simulink model "ALL_JP360_DBW_V6_5_1103"  (R2022a)
settings: Solver=FixedStepAuto  StartTime=0.0  StopTime=inf  FixedStep=0.01  RelTol=1e-3  EnableMultiTasking=on
model workspace (MAT data in the model file):
  g = 9.8
undefined symbols (not defined in the file or in its folder): canChannel, delta_v_p, IPM_Line_C0, IPM_Line_C1, IPM_Line_C2, IPM_Line_C3, M, M_p, MRR_ObjDistX, MRR_ObjDistY, MRR_ObjFusionCamID, MRR_ObjFusionSig, MRR_ObjID, MRR_ObjRelVelX, MRR_ObjRelVelY, MRR_ObjType, MRR_ObjUpdFlg, none, obj_vaild, untracktime, V, videoinput
libraries: canfdmsglib x230, canfdlib x76, slpidlib x24, simulink x18, dspstat3 x14, ctrlSharedLib x1, simulink_extras x1, imaqlib x1, realtime_pacer_lib x1, dspvision x1, visionsinks x1
(part 42 of 55)

== system ALL_JP360_DBW_V6_5_1103/MsgFromCAN/VR_ADCU_MsgFromCAN/VR_ADCU_IPM_Line_01_0x640 ==
  VR_ADCU_IPM_Line_01_0x640FromInData : Inport  OutDataTypeStr=Bus:CAN_FD_MESSAGE_BUS
  Bus Creator : BusCreator  Inputs=12  OutDataTypeStr=Bus:VR_ADCU_IPM_Line_01_0x640  NonVirtualBus=on
  CAN FD Unpack : canfdmsglib/CAN FD Unpack  CANdbFile=HiFire_T360_P789_1R1V_Pri_Matrix_CAN_V2.3_20220810.dbc  MsgList=(none)  MsgName=IPM_Line_01_0x640  ProtocolMode=CAN FD  MsgIDType=Standard (11-bit identifier)  MsgIdentifier=1600  MsgLength=20  SignalInfo={'IPM_Line01_BlockCounter','90','11','BE','unsigned','Standard','0','1','0','0','2047';'IPM_Line01_C0','115','13','BE','unsigned','Standard','0','0.0039062','-16','-16','15.9961';'IPM_Line01_C1','61','13','BE','unsigned','Standard','0','0.00048828','-1.6','-1.6','1.6002';'IPM_Line01_C2','65','12','BE','unsigned','Standard','0','1.5259e-05','-0.031243','-0.031243','0.031206';'IPM_Line01_C3','85','12','BE','unsigned','Standard','0','3.8147e-06','-0.0078125','-0.0078125','0.0078087';'IPM_Line01_Checksum','152','16','BE','unsigned','Standard','0','1','0','0','65535';'IPM_Line01_ColorClass','12','3','BE','unsigned','Standard','0','1','0','0','7';'IPM_Line01_Existence_Probability','96','8','BE','unsigned','Standard','0','0.01','0','0','1';'IPM_Line01_MsgCounter','136','4','BE','unsigned','Standard','0','1','0','0','15';'IPM_Line01_Type','15','5','BE','unsigned','Standard','0','1','0','0','31';'IPM_Line01_ViewRangeEnd','37','10','BE','unsigned','Standard','0','0.25','0','0','255.75';'IPM_Line01_ViewRangeStart','31','13','BE','unsigned','Standard','0','0.025','0','0','204.775'}  IDPort=off  TimestampPort=off  ErrorPort=off  RemotePort=off  LengthPort=off  StatusPort=off  BRSPort=off  ESIPort=off  DLCPort=off  ApplyMinMax=off
      settings: SourceProductBaseCode=ME,XP,VN  DataFormat=CANdb specified signals
  Data Type Conversion1 : DataTypeConversion  OutDataTypeStr=int16  SaturateOnIntegerOverflow=off  RndMeth=Floor
  Data Type Conversion10 : DataTypeConversion  OutDataTypeStr=int8  SaturateOnIntegerOverflow=off  RndMeth=Floor
  Data Type Conversion{2..5,8,11..12} (7 alike) : DataTypeConversion  OutDataTypeStr=single  SaturateOnIntegerOverflow=off  RndMeth=Floor
  Data Type Conversion6 : DataTypeConversion  OutDataTypeStr=uint16  SaturateOnIntegerOverflow=off  RndMeth=Floor
  Data Type Conversion7 : DataTypeConversion  OutDataTypeStr=int8  SaturateOnIntegerOverflow=off  RndMeth=Floor
  Data Type Conversion9 : DataTypeConversion  OutDataTypeStr=int8  SaturateOnIntegerOverflow=off  RndMeth=Floor
  VR_ADCU_IPM_Line_01_0x640FromOutData : Outport  OutDataTypeStr=Bus:VR_ADCU_IPM_Line_01_0x640
  wires:
  CAN FD Unpack/1 -> Data Type Conversion1/1
  CAN FD Unpack/2 -> Data Type Conversion2/1
  CAN FD Unpack/3 -> Data Type Conversion3/1
  CAN FD Unpack/4 -> Data Type Conversion4/1
  CAN FD Unpack/5 -> Data Type Conversion5/1
  CAN FD Unpack/6 -> Data Type Conversion6/1
  CAN FD Unpack/7 -> Data Type Conversion7/1
  CAN FD Unpack/8 -> Data Type Conversion8/1
  CAN FD Unpack/9 -> Data Type Conversion9/1
  CAN FD Unpack/10 -> Data Type Conversion10/1
  CAN FD Unpack/11 -> Data Type Conversion11/1
  CAN FD Unpack/12 -> Data Type Conversion12/1
  Data Type Conversion1/1 -> Bus Creator/1  "IPM_Line01_BlockCounter"
  Data Type Conversion2/1 -> Bus Creator/2  "IPM_Line01_C0"
  Data Type Conversion3/1 -> Bus Creator/3  "IPM_Line01_C1"
  Data Type Conversion4/1 -> Bus Creator/4  "IPM_Line01_C2"
  Data Type Conversion5/1 -> Bus Creator/5  "IPM_Line01_C3"
  Data Type Conversion6/1 -> Bus Creator/6  "IPM_Line01_Checksum"
  Data Type Conversion7/1 -> Bus Creator/7  "IPM_Line01_ColorClass"
  Data Type Conversion8/1 -> Bus Creator/8  "IPM_Line01_Existence_Probability"
  Data Type Conversion9/1 -> Bus Creator/9  "IPM_Line01_MsgCounter"
  Data Type Conversion10/1 -> Bus Creator/10  "IPM_Line01_Type"
  Data Type Conversion11/1 -> Bus Creator/11  "IPM_Line01_ViewRangeEnd"
  Data Type Conversion12/1 -> Bus Creator/12  "IPM_Line01_ViewRangeStart"
  Bus Creator/1 -> VR_ADCU_IPM_Line_01_0x640FromOutData/1  "VR_ADCU_IPM_Line_01_0x640FromOutData"
  VR_ADCU_IPM_Line_01_0x640FromInData/1 -> CAN FD Unpack/1  "VR_ADCU_IPM_Line_01_0x640FromInData"

== system ALL_JP360_DBW_V6_5_1103/MsgFromCAN/VR_ADCU_MsgFromCAN/VR_ADCU_IPM_Line_02_0x641 ==
  VR_ADCU_IPM_Line_02_0x641FromInData : Inport  OutDataTypeStr=Bus:CAN_FD_MESSAGE_BUS
  Bus Creator : BusCreator  Inputs=12  OutDataTypeStr=Bus:VR_ADCU_IPM_Line_02_0x641  NonVirtualBus=on
  CAN FD Unpack : canfdmsglib/CAN FD Unpack  CANdbFile=HiFire_T360_P789_1R1V_Pri_Matrix_CAN_V2.3_20220810.dbc  MsgList=(none)  MsgName=IPM_Line_02_0x641  ProtocolMode=CAN FD  MsgIDType=Standard (11-bit identifier)  MsgIdentifier=1601  MsgLength=20  SignalInfo={'IPM_Line02_BlockCounter','90','11','BE','unsigned','Standard','0','1','0','0','2047';'IPM_Line02_C0','115','13','BE','unsigned','Standard','0','0.0039062','-16','-16','15.9961';'IPM_Line02_C1','61','13','BE','unsigned','Standard','0','0.00048828','-1.6','-1.6','1.6002';'IPM_Line02_C2','65','12','BE','unsigned','Standard','0','1.5259e-05','-0.031243','-0.031243','0.031206';'IPM_Line02_C3','85','12','BE','unsigned','Standard','0','3.8147e-06','-0.0078125','-0.0078125','0.0078087';'IPM_Line02_Checksum','152','16','BE','unsigned','Standard','0','1','0','0','65535';'IPM_Line02_ColorClass','12','3','BE','unsigned','Standard','0','1','0','0','7';'IPM_Line02_Existence_Probability','96','8','BE','unsigned','Standard','0','0.01','0','0','1';'IPM_Line02_MsgCounter','136','4','BE','unsigned','Standard','0','1','0','0','15';'IPM_Line02_Type','15','5','BE','unsigned','Standard','0','1','0','0','31';'IPM_Line02_ViewRangeEnd','37','10','BE','unsigned','Standard','0','0.25','0','0','255.75';'IPM_Line02_ViewRangeStart','31','13','BE','unsigned','Standard','0','0.025','0','0','204.775'}  IDPort=off  TimestampPort=off  ErrorPort=off  RemotePort=off  LengthPort=off  StatusPort=off  BRSPort=off  ESIPort=off  DLCPort=off  ApplyMinMax=off
      settings: SourceProductBaseCode=ME,XP,VN  DataFormat=CANdb specified signals
  Data Type Conversion1 : DataTypeConversion  OutDataTypeStr=int16  SaturateOnIntegerOverflow=off  RndMeth=Floor
  Data Type Conversion10 : DataTypeConversion  OutDataTypeStr=int8  SaturateOnIntegerOverflow=off  RndMeth=Floor
  Data Type Conversion{2..5,8,11..12} (7 alike) : DataTypeConversion  OutDataTypeStr=single  SaturateOnIntegerOverflow=off  RndMeth=Floor
  Data Type Conversion6 : DataTypeConversion  OutDataTypeStr=uint16  SaturateOnIntegerOverflow=off  RndMeth=Floor
  Data Type Conversion7 : DataTypeConversion  OutDataTypeStr=int8  SaturateOnIntegerOverflow=off  RndMeth=Floor
  Data Type Conversion9 : DataTypeConversion  OutDataTypeStr=int8  SaturateOnIntegerOverflow=off  RndMeth=Floor
  VR_ADCU_IPM_Line_02_0x641FromOutData : Outport  OutDataTypeStr=Bus:VR_ADCU_IPM_Line_02_0x641
  wires:
  CAN FD Unpack/1 -> Data Type Conversion1/1
  CAN FD Unpack/2 -> Data Type Conversion2/1
  CAN FD Unpack/3 -> Data Type Conversion3/1
  CAN FD Unpack/4 -> Data Type Conversion4/1
  CAN FD Unpack/5 -> Data Type Conversion5/1
  CAN FD Unpack/6 -> Data Type Conversion6/1
  CAN FD Unpack/7 -> Data Type Conversion7/1
  CAN FD Unpack/8 -> Data Type Conversion8/1
  CAN FD Unpack/9 -> Data Type Conversion9/1
  CAN FD Unpack/10 -> Data Type Conversion10/1
  CAN FD Unpack/11 -> Data Type Conversion11/1
  CAN FD Unpack/12 -> Data Type Conversion12/1
  Data Type Conversion1/1 -> Bus Creator/1  "IPM_Line02_BlockCounter"
  Data Type Conversion2/1 -> Bus Creator/2  "IPM_Line02_C0"
  Data Type Conversion3/1 -> Bus Creator/3  "IPM_Line02_C1"
  Data Type Conversion4/1 -> Bus Creator/4  "IPM_Line02_C2"
  Data Type Conversion5/1 -> Bus Creator/5  "IPM_Line02_C3"
  Data Type Conversion6/1 -> Bus Creator/6  "IPM_Line02_Checksum"
  Data Type Conversion7/1 -> Bus Creator/7  "IPM_Line02_ColorClass"
  Data Type Conversion8/1 -> Bus Creator/8  "IPM_Line02_Existence_Probability"
  Data Type Conversion9/1 -> Bus Creator/9  "IPM_Line02_MsgCounter"
  Data Type Conversion10/1 -> Bus Creator/10  "IPM_Line02_Type"
  Data Type Conversion11/1 -> Bus Creator/11  "IPM_Line02_ViewRangeEnd"
  Data Type Conversion12/1 -> Bus Creator/12  "IPM_Line02_ViewRangeStart"
  Bus Creator/1 -> VR_ADCU_IPM_Line_02_0x641FromOutData/1  "VR_ADCU_IPM_Line_02_0x641FromOutData"
  VR_ADCU_IPM_Line_02_0x641FromInData/1 -> CAN FD Unpack/1  "VR_ADCU_IPM_Line_02_0x641FromInData"

== system ALL_JP360_DBW_V6_5_1103/MsgFromCAN/VR_ADCU_MsgFromCAN/VR_ADCU_IPM_Line_03_0x642 ==
  VR_ADCU_IPM_Line_03_0x642FromInData : Inport  OutDataTypeStr=Bus:CAN_FD_MESSAGE_BUS
  Bus Creator : BusCreator  Inputs=12  OutDataTypeStr=Bus:VR_ADCU_IPM_Line_03_0x642  NonVirtualBus=on
  CAN FD Unpack : canfdmsglib/CAN FD Unpack  CANdbFile=HiFire_T360_P789_1R1V_Pri_Matrix_CAN_V2.3_20220810.dbc  MsgList=(none)  MsgName=IPM_Line_03_0x642  ProtocolMode=CAN FD  MsgIDType=Standard (11-bit identifier)  MsgIdentifier=1602  MsgLength=20  SignalInfo={'IPM_Line03_BlockCounter','90','11','BE','unsigned','Standard','0','1','0','0','2047';'IPM_Line03_C0','115','13','BE','unsigned','Standard','0','0.0039062','-16','-16','15.9961';'IPM_Line03_C1','61','13','BE','unsigned','Standard','0','0.00048828','-1.6','-1.6','1.6002';'IPM_Line03_C2','65','12','BE','unsigned','Standard','0','1.5259e-05','-0.031243','-0.031243','0.031206';'IPM_Line03_C3','85','12','BE','unsigned','Standard','0','3.8147e-06','-0.0078125','-0.0078125','0.0078087';'IPM_Line03_Checksum','152','16','BE','unsigned','Standard','0','1','0','0','65535';'IPM_Line03_ColorClass','12','3','BE','unsigned','Standard','0','1','0','0','7';'IPM_Line03_Existence_Probability','96','8','BE','unsigned','Standard','0','0.01','0','0','1';'IPM_Line03_MsgCounter','136','4','BE','unsigned','Standard','0','1','0','0','15';'IPM_Line03_Type','15','5','BE','unsigned','Standard','0','1','0','0','31';'IPM_Line03_ViewRangeEnd','37','10','BE','unsigned','Standard','0','0.25','0','0','255.75';'IPM_Line03_ViewRangeStart','31','13','BE','unsigned','Standard','0','0.025','0','0','204.775'}  IDPort=off  TimestampPort=off  ErrorPort=off  RemotePort=off  LengthPort=off  StatusPort=off  BRSPort=off  ESIPort=off  DLCPort=off  ApplyMinMax=off
      settings: SourceProductBaseCode=ME,XP,VN  DataFormat=CANdb specified signals
  Data Type Conversion1 : DataTypeConversion  OutDataTypeStr=int16  SaturateOnIntegerOverflow=off  RndMeth=Floor
  Data Type Conversion10 : DataTypeConversion  OutDataTypeStr=int8  SaturateOnIntegerOverflow=off  RndMeth=Floor
  Data Type Conversion{2..5,8,11..12} (7 alike) : DataTypeConversion  OutDataTypeStr=single  SaturateOnIntegerOverflow=off  RndMeth=Floor
  Data Type Conversion6 : DataTypeConversion  OutDataTypeStr=uint16  SaturateOnIntegerOverflow=off  RndMeth=Floor
  Data Type Conversion7 : DataTypeConversion  OutDataTypeStr=int8  SaturateOnIntegerOverflow=off  RndMeth=Floor
  Data Type Conversion9 : DataTypeConversion  OutDataTypeStr=int8  SaturateOnIntegerOverflow=off  RndMeth=Floor
  VR_ADCU_IPM_Line_03_0x642FromOutData : Outport  OutDataTypeStr=Bus:VR_ADCU_IPM_Line_03_0x642
  wires:
  CAN FD Unpack/1 -> Data Type Conversion1/1
  CAN FD Unpack/2 -> Data Type Conversion2/1
  CAN FD Unpack/3 -> Data Type Conversion3/1
  CAN FD Unpack/4 -> Data Type Conversion4/1
  CAN FD Unpack/5 -> Data Type Conversion5/1
  CAN FD Unpack/6 -> Data Type Conversion6/1
  CAN FD Unpack/7 -> Data Type Conversion7/1
  CAN FD Unpack/8 -> Data Type Conversion8/1
  CAN FD Unpack/9 -> Data Type Conversion9/1
  CAN FD Unpack/10 -> Data Type Conversion10/1
  CAN FD Unpack/11 -> Data Type Conversion11/1
  CAN FD Unpack/12 -> Data Type Conversion12/1
  Data Type Conversion1/1 -> Bus Creator/1  "IPM_Line03_BlockCounter"
  Data Type Conversion2/1 -> Bus Creator/2  "IPM_Line03_C0"
  Data Type Conversion3/1 -> Bus Creator/3  "IPM_Line03_C1"
  Data Type Conversion4/1 -> Bus Creator/4  "IPM_Line03_C2"
  Data Type Conversion5/1 -> Bus Creator/5  "IPM_Line03_C3"
  Data Type Conversion6/1 -> Bus Creator/6  "IPM_Line03_Checksum"
  Data Type Conversion7/1 -> Bus Creator/7  "IPM_Line03_ColorClass"
  Data Type Conversion8/1 -> Bus Creator/8  "IPM_Line03_Existence_Probability"
  Data Type Conversion9/1 -> Bus Creator/9  "IPM_Line03_MsgCounter"
  Data Type Conversion10/1 -> Bus Creator/10  "IPM_Line03_Type"
  Data Type Conversion11/1 -> Bus Creator/11  "IPM_Line03_ViewRangeEnd"
  Data Type Conversion12/1 -> Bus Creator/12  "IPM_Line03_ViewRangeStart"
  Bus Creator/1 -> VR_ADCU_IPM_Line_03_0x642FromOutData/1  "VR_ADCU_IPM_Line_03_0x642FromOutData"
  VR_ADCU_IPM_Line_03_0x642FromInData/1 -> CAN FD Unpack/1  "VR_ADCU_IPM_Line_03_0x642FromInData"

== system ALL_JP360_DBW_V6_5_1103/MsgFromCAN/VR_ADCU_MsgFromCAN/VR_ADCU_IPM_Line_04_0x643 ==
  VR_ADCU_IPM_Line_04_0x643FromInData : Inport  OutDataTypeStr=Bus:CAN_FD_MESSAGE_BUS
  Bus Creator : BusCreator  Inputs=12  OutDataTypeStr=Bus:VR_ADCU_IPM_Line_04_0x643  NonVirtualBus=on
  CAN FD Unpack : canfdmsglib/CAN FD Unpack  CANdbFile=HiFire_T360_P789_1R1V_Pri_Matrix_CAN_V2.3_20220810.dbc  MsgList=(none)  MsgName=IPM_Line_04_0x643  ProtocolMode=CAN FD  MsgIDType=Standard (11-bit identifier)  MsgIdentifier=1603  MsgLength=20  SignalInfo={'IPM_Line04_BlockCounter','90','11','BE','unsigned','Standard','0','1','0','0','2047';'IPM_Line04_C0','115','13','BE','unsigned','Standard','0','0.0039062','-16','-16','15.9961';'IPM_Line04_C1','61','13','BE','unsigned','Standard','0','0.00048828','-1.6','-1.6','1.6002';'IPM_Line04_C2','65','12','BE','unsigned','Standard','0','1.5259e-05','-0.031243','-0.031243','0.031206';'IPM_Line04_C3','85','12','BE','unsigned','Standard','0','3.8147e-06','-0.0078125','-0.0078125','0.0078087';'IPM_Line04_Checksum','152','16','BE','unsigned','Standard','0','1','0','0','65535';'IPM_Line04_ColorClass','12','3','BE','unsigned','Standard','0','1','0','0','7';'IPM_Line04_Existence_Probability','96','8','BE','unsigned','Standard','0','0.01','0','0','1';'IPM_Line04_MsgCounter','136','4','BE','unsigned','Standard','0','1','0','0','15';'IPM_Line04_Type','15','5','BE','unsigned','Standard','0','1','0','0','31';'IPM_Line04_ViewRangeEnd','37','10','BE','unsigned','Standard','0','0.25','0','0','255.75';'IPM_Line04_ViewRangeStart','31','13','BE','unsigned','Standard','0','0.025','0','0','204.775'}  IDPort=off  TimestampPort=off  ErrorPort=off  RemotePort=off  LengthPort=off  StatusPort=off  BRSPort=off  ESIPort=off  DLCPort=off  ApplyMinMax=off
      settings: SourceProductBaseCode=ME,XP,VN  DataFormat=CANdb specified signals
  Data Type Conversion1 : DataTypeConversion  OutDataTypeStr=int16  SaturateOnIntegerOverflow=off  RndMeth=Floor
  Data Type Conversion10 : DataTypeConversion  OutDataTypeStr=int8  SaturateOnIntegerOverflow=off  RndMeth=Floor
  Data Type Conversion{2..5,8,11..12} (7 alike) : DataTypeConversion  OutDataTypeStr=single  SaturateOnIntegerOverflow=off  RndMeth=Floor
  Data Type Conversion6 : DataTypeConversion  OutDataTypeStr=uint16  SaturateOnIntegerOverflow=off  RndMeth=Floor
  Data Type Conversion7 : DataTypeConversion  OutDataTypeStr=int8  SaturateOnIntegerOverflow=off  RndMeth=Floor
  Data Type Conversion9 : DataTypeConversion  OutDataTypeStr=int8  SaturateOnIntegerOverflow=off  RndMeth=Floor
  VR_ADCU_IPM_Line_04_0x643FromOutData : Outport  OutDataTypeStr=Bus:VR_ADCU_IPM_Line_04_0x643
  wires:
  CAN FD Unpack/1 -> Data Type Conversion1/1
  CAN FD Unpack/2 -> Data Type Conversion2/1
  CAN FD Unpack/3 -> Data Type Conversion3/1
  CAN FD Unpack/4 -> Data Type Conversion4/1
  CAN FD Unpack/5 -> Data Type Conversion5/1
  CAN FD Unpack/6 -> Data Type Conversion6/1
  CAN FD Unpack/7 -> Data Type Conversion7/1
  CAN FD Unpack/8 -> Data Type Conversion8/1
  CAN FD Unpack/9 -> Data Type Conversion9/1
  CAN FD Unpack/10 -> Data Type Conversion10/1
  CAN FD Unpack/11 -> Data Type Conversion11/1
  CAN FD Unpack/12 -> Data Type Conversion12/1
  Data Type Conversion1/1 -> Bus Creator/1  "IPM_Line04_BlockCounter"
  Data Type Conversion2/1 -> Bus Creator/2  "IPM_Line04_C0"
  Data Type Conversion3/1 -> Bus Creator/3  "IPM_Line04_C1"
  Data Type Conversion4/1 -> Bus Creator/4  "IPM_Line04_C2"
  Data Type Conversion5/1 -> Bus Creator/5  "IPM_Line04_C3"
  Data Type Conversion6/1 -> Bus Creator/6  "IPM_Line04_Checksum"
  Data Type Conversion7/1 -> Bus Creator/7  "IPM_Line04_ColorClass"
  Data Type Conversion8/1 -> Bus Creator/8  "IPM_Line04_Existence_Probability"
  Data Type Conversion9/1 -> Bus Creator/9  "IPM_Line04_MsgCounter"
  Data Type Conversion10/1 -> Bus Creator/10  "IPM_Line04_Type"
  Data Type Conversion11/1 -> Bus Creator/11  "IPM_Line04_ViewRangeEnd"
  Data Type Conversion12/1 -> Bus Creator/12  "IPM_Line04_ViewRangeStart"
  Bus Creator/1 -> VR_ADCU_IPM_Line_04_0x643FromOutData/1  "VR_ADCU_IPM_Line_04_0x643FromOutData"
  VR_ADCU_IPM_Line_04_0x643FromInData/1 -> CAN FD Unpack/1  "VR_ADCU_IPM_Line_04_0x643FromInData"

== system ALL_JP360_DBW_V6_5_1103/MsgFromCAN/VR_ADCU_MsgFromCAN/VR_ADCU_IPM_Line_05_0x644 ==
  VR_ADCU_IPM_Line_05_0x644FromInData : Inport  OutDataTypeStr=Bus:CAN_FD_MESSAGE_BUS
  Bus Creator : BusCreator  Inputs=12  OutDataTypeStr=Bus:VR_ADCU_IPM_Line_05_0x644  NonVirtualBus=on
  CAN FD Unpack : canfdmsglib/CAN FD Unpack  CANdbFile=HiFire_T360_P789_1R1V_Pri_Matrix_CAN_V2.3_20220810.dbc  MsgList=(none)  MsgName=IPM_Line_05_0x644  ProtocolMode=CAN FD  MsgIDType=Standard (11-bit identifier)  MsgIdentifier=1604  MsgLength=20  SignalInfo={'IPM_Line05_BlockCounter','90','11','BE','unsigned','Standard','0','1','0','0','2047';'IPM_Line05_C0','115','13','BE','unsigned','Standard','0','0.0039062','-16','-16','15.9961';'IPM_Line05_C1','61','13','BE','unsigned','Standard','0','0.00048828','-1.6','-1.6','1.6002';'IPM_Line05_C2','65','12','BE','unsigned','Standard','0','1.5259e-05','-0.031243','-0.031243','0.031206';'IPM_Line05_C3','85','12','BE','unsigned','Standard','0','3.8147e-06','-0.0078125','-0.0078125','0.0078087';'IPM_Line05_Checksum','152','16','BE','unsigned','Standard','0','1','0','0','65535';'IPM_Line05_ColorClass','12','3','BE','unsigned','Standard','0','1','0','0','7';'IPM_Line05_Existence_Probability','96','8','BE','unsigned','Standard','0','0.01','0','0','1';'IPM_Line05_MsgCounter','136','4','BE','unsigned','Standard','0','1','0','0','15';'IPM_Line05_Type','15','5','BE','unsigned','Standard','0','1','0','0','31';'IPM_Line05_ViewRangeEnd','37','10','BE','unsigned','Standard','0','0.25','0','0','255.75';'IPM_Line05_ViewRangeStart','31','13','BE','unsigned','Standard','0','0.025','0','0','204.775'}  IDPort=off  TimestampPort=off  ErrorPort=off  RemotePort=off  LengthPort=off  StatusPort=off  BRSPort=off  ESIPort=off  DLCPort=off  ApplyMinMax=off
      settings: SourceProductBaseCode=ME,XP,VN  DataFormat=CANdb specified signals
  Data Type Conversion1 : DataTypeConversion  OutDataTypeStr=int16  SaturateOnIntegerOverflow=off  RndMeth=Floor
  Data Type Conversion10 : DataTypeConversion  OutDataTypeStr=int8  SaturateOnIntegerOverflow=off  RndMeth=Floor
  Data Type Conversion{2..5,8,11..12} (7 alike) : DataTypeConversion  OutDataTypeStr=single  SaturateOnIntegerOverflow=off  RndMeth=Floor
  Data Type Conversion6 : DataTypeConversion  OutDataTypeStr=uint16  SaturateOnIntegerOverflow=off  RndMeth=Floor
  Data Type Conversion7 : DataTypeConversion  OutDataTypeStr=int8  SaturateOnIntegerOverflow=off  RndMeth=Floor
  Data Type Conversion9 : DataTypeConversion  OutDataTypeStr=int8  SaturateOnIntegerOverflow=off  RndMeth=Floor
  VR_ADCU_IPM_Line_05_0x644FromOutData : Outport  OutDataTypeStr=Bus:VR_ADCU_IPM_Line_05_0x644
  wires:
  CAN FD Unpack/1 -> Data Type Conversion1/1
  CAN FD Unpack/2 -> Data Type Conversion2/1
  CAN FD Unpack/3 -> Data Type Conversion3/1
  CAN FD Unpack/4 -> Data Type Conversion4/1
  CAN FD Unpack/5 -> Data Type Conversion5/1
  CAN FD Unpack/6 -> Data Type Conversion6/1
  CAN FD Unpack/7 -> Data Type Conversion7/1
  CAN FD Unpack/8 -> Data Type Conversion8/1
  CAN FD Unpack/9 -> Data Type Conversion9/1
  CAN FD Unpack/10 -> Data Type Conversion10/1
  CAN FD Unpack/11 -> Data Type Conversion11/1
  CAN FD Unpack/12 -> Data Type Conversion12/1
  Data Type Conversion1/1 -> Bus Creator/1  "IPM_Line05_BlockCounter"
  Data Type Conversion2/1 -> Bus Creator/2  "IPM_Line05_C0"
  Data Type Conversion3/1 -> Bus Creator/3  "IPM_Line05_C1"
  Data Type Conversion4/1 -> Bus Creator/4  "IPM_Line05_C2"
  Data Type Conversion5/1 -> Bus Creator/5  "IPM_Line05_C3"
  Data Type Conversion6/1 -> Bus Creator/6  "IPM_Line05_Checksum"
  Data Type Conversion7/1 -> Bus Creator/7  "IPM_Line05_ColorClass"
  Data Type Conversion8/1 -> Bus Creator/8  "IPM_Line05_Existence_Probability"
  Data Type Conversion9/1 -> Bus Creator/9  "IPM_Line05_MsgCounter"
  Data Type Conversion10/1 -> Bus Creator/10  "IPM_Line05_Type"
  Data Type Conversion11/1 -> Bus Creator/11  "IPM_Line05_ViewRangeEnd"
  Data Type Conversion12/1 -> Bus Creator/12  "IPM_Line05_ViewRangeStart"
  Bus Creator/1 -> VR_ADCU_IPM_Line_05_0x644FromOutData/1  "VR_ADCU_IPM_Line_05_0x644FromOutData"
  VR_ADCU_IPM_Line_05_0x644FromInData/1 -> CAN FD Unpack/1  "VR_ADCU_IPM_Line_05_0x644FromInData"

== system ALL_JP360_DBW_V6_5_1103/MsgFromCAN/VR_ADCU_MsgFromCAN/VR_ADCU_IPM_Line_06_0x645 ==
  VR_ADCU_IPM_Line_06_0x645FromInData : Inport  OutDataTypeStr=Bus:CAN_FD_MESSAGE_BUS
  Bus Creator : BusCreator  Inputs=12  OutDataTypeStr=Bus:VR_ADCU_IPM_Line_06_0x645  NonVirtualBus=on
  CAN FD Unpack : canfdmsglib/CAN FD Unpack  CANdbFile=HiFire_T360_P789_1R1V_Pri_Matrix_CAN_V2.3_20220810.dbc  MsgList=(none)  MsgName=IPM_Line_06_0x645  ProtocolMode=CAN FD  MsgIDType=Standard (11-bit identifier)  MsgIdentifier=1605  MsgLength=20  SignalInfo={'IPM_Line06_BlockCounter','90','11','BE','unsigned','Standard','0','1','0','0','2047';'IPM_Line06_C0','115','13','BE','unsigned','Standard','0','0.0039062','-16','-16','15.9961';'IPM_Line06_C1','61','13','BE','unsigned','Standard','0','0.00048828','-1.6','-1.6','1.6002';'IPM_Line06_C2','65','12','BE','unsigned','Standard','0','1.5259e-05','-0.031243','-0.031243','0.031206';'IPM_Line06_C3','85','12','BE','unsigned','Standard','0','3.8147e-06','-0.0078125','-0.0078125','0.0078087';'IPM_Line06_Checksum','152','16','BE','unsigned','Standard','0','1','0','0','65535';'IPM_Line06_ColorClass','12','3','BE','unsigned','Standard','0','1','0','0','7';'IPM_Line06_Existence_Probability','96','8','BE','unsigned','Standard','0','0.01','0','0','1';'IPM_Line06_MsgCounter','136','4','BE','unsigned','Standard','0','1','0','0','15';'IPM_Line06_Type','15','5','BE','unsigned','Standard','0','1','0','0','31';'IPM_Line06_ViewRangeEnd','37','10','BE','unsigned','Standard','0','0.25','0','0','255.75';'IPM_Line06_ViewRangeStart','31','13','BE','unsigned','Standard','0','0.025','0','0','204.775'}  IDPort=off  TimestampPort=off  ErrorPort=off  RemotePort=off  LengthPort=off  StatusPort=off  BRSPort=off  ESIPort=off  DLCPort=off  ApplyMinMax=off
      settings: SourceProductBaseCode=ME,XP,VN  DataFormat=CANdb specified signals
  Data Type Conversion1 : DataTypeConversion  OutDataTypeStr=int16  SaturateOnIntegerOverflow=off  RndMeth=Floor
  Data Type Conversion10 : DataTypeConversion  OutDataTypeStr=int8  SaturateOnIntegerOverflow=off  RndMeth=Floor
  Data Type Conversion{2..5,8,11..12} (7 alike) : DataTypeConversion  OutDataTypeStr=single  SaturateOnIntegerOverflow=off  RndMeth=Floor
  Data Type Conversion6 : DataTypeConversion  OutDataTypeStr=uint16  SaturateOnIntegerOverflow=off  RndMeth=Floor
  Data Type Conversion7 : DataTypeConversion  OutDataTypeStr=int8  SaturateOnIntegerOverflow=off  RndMeth=Floor
  Data Type Conversion9 : DataTypeConversion  OutDataTypeStr=int8  SaturateOnIntegerOverflow=off  RndMeth=Floor
  VR_ADCU_IPM_Line_06_0x645FromOutData : Outport  OutDataTypeStr=Bus:VR_ADCU_IPM_Line_06_0x645
  wires:
  CAN FD Unpack/1 -> Data Type Conversion1/1
  CAN FD Unpack/2 -> Data Type Conversion2/1
  CAN FD Unpack/3 -> Data Type Conversion3/1
  CAN FD Unpack/4 -> Data Type Conversion4/1
  CAN FD Unpack/5 -> Data Type Conversion5/1
  CAN FD Unpack/6 -> Data Type Conversion6/1
  CAN FD Unpack/7 -> Data Type Conversion7/1
  CAN FD Unpack/8 -> Data Type Conversion8/1
  CAN FD Unpack/9 -> Data Type Conversion9/1
  CAN FD Unpack/10 -> Data Type Conversion10/1
  CAN FD Unpack/11 -> Data Type Conversion11/1
  CAN FD Unpack/12 -> Data Type Conversion12/1
  Data Type Conversion1/1 -> Bus Creator/1  "IPM_Line06_BlockCounter"
  Data Type Conversion2/1 -> Bus Creator/2  "IPM_Line06_C0"
  Data Type Conversion3/1 -> Bus Creator/3  "IPM_Line06_C1"
  Data Type Conversion4/1 -> Bus Creator/4  "IPM_Line06_C2"
  Data Type Conversion5/1 -> Bus Creator/5  "IPM_Line06_C3"
  Data Type Conversion6/1 -> Bus Creator/6  "IPM_Line06_Checksum"
  Data Type Conversion7/1 -> Bus Creator/7  "IPM_Line06_ColorClass"
  Data Type Conversion8/1 -> Bus Creator/8  "IPM_Line06_Existence_Probability"
  Data Type Conversion9/1 -> Bus Creator/9  "IPM_Line06_MsgCounter"
  Data Type Conversion10/1 -> Bus Creator/10  "IPM_Line06_Type"
  Data Type Conversion11/1 -> Bus Creator/11  "IPM_Line06_ViewRangeEnd"
  Data Type Conversion12/1 -> Bus Creator/12  "IPM_Line06_ViewRangeStart"
  Bus Creator/1 -> VR_ADCU_IPM_Line_06_0x645FromOutData/1  "VR_ADCU_IPM_Line_06_0x645FromOutData"
  VR_ADCU_IPM_Line_06_0x645FromInData/1 -> CAN FD Unpack/1  "VR_ADCU_IPM_Line_06_0x645FromInData"

== system ALL_JP360_DBW_V6_5_1103/MsgFromCAN/VR_ADCU_MsgFromCAN/VR_ADCU_IPM_ObjHeader_0x630 ==
  VR_ADCU_IPM_ObjHeader_0x630FromInData : Inport  OutDataTypeStr=Bus:CAN_FD_MESSAGE_BUS
  Bus Creator : BusCreator  Inputs=7  OutDataTypeStr=Bus:VR_ADCU_IPM_ObjHeader_0x630  NonVirtualBus=on
  CAN FD Unpack : canfdmsglib/CAN FD Unpack  CANdbFile=HiFire_T360_P789_1R1V_Pri_Matrix_CAN_V2.3_20220810.dbc  MsgList=(none)  MsgName=IPM_ObjHeader_0x630  ProtocolMode=CAN FD  MsgIDType=Standard (11-bit identifier)  MsgIdentifier=1584  MsgLength=20  SignalInfo={'IPM_ObjHeaderBlockCounter','85','11','BE','unsigned','Standard','0','1','0','0','2047';'IPM_ObjHeader_Checksum','152','16','BE','unsigned','Standard','0','1','0','0','65535';'IPM_ObjHeader_MsgCounter','136','4','BE','unsigned','Standard','0','1','0','0','15';'IPM_Obj_TimeStampStatus','88','8','BE','unsigned','Standard','0','1','0','0','255';'IPM_Obj_TimeStamp_Nsec','66','30','BE','unsigned','Standard','0','1','0','0','1073741823';'IPM_Obj_TimeStamp_sec','32','32','BE','unsigned','Standard','0','1','0','0','4294967295';'IPM_SensorState','5','3','BE','unsigned','Standard','0','1','0','0','7'}  IDPort=off  TimestampPort=off  ErrorPort=off  RemotePort=off  LengthPort=off  StatusPort=off  BRSPort=off  ESIPort=off  DLCPort=off  ApplyMinMax=off
      settings: SourceProductBaseCode=ME,XP,VN  DataFormat=CANdb specified signals
  Data Type Conversion1 : DataTypeConversion  OutDataTypeStr=int16  SaturateOnIntegerOverflow=off  RndMeth=Floor
  Data Type Conversion2 : DataTypeConversion  OutDataTypeStr=uint16  SaturateOnIntegerOverflow=off  RndMeth=Floor
  Data Type Conversion3 : DataTypeConversion  OutDataTypeStr=int8  SaturateOnIntegerOverflow=off  RndMeth=Floor
  Data Type Conversion4 : DataTypeConversion  OutDataTypeStr=uint8  SaturateOnIntegerOverflow=off  RndMeth=Floor
  Data Type Conversion5 : DataTypeConversion  OutDataTypeStr=int32  SaturateOnIntegerOverflow=off  RndMeth=Floor
  Data Type Conversion6 : DataTypeConversion  OutDataTypeStr=uint32  SaturateOnIntegerOverflow=off  RndMeth=Floor
  Data Type Conversion7 : DataTypeConversion  OutDataTypeStr=int8  SaturateOnIntegerOverflow=off  RndMeth=Floor
  VR_ADCU_IPM_ObjHeader_0x630FromOutData : Outport  OutDataTypeStr=Bus:VR_ADCU_IPM_ObjHeader_0x630
  wires:
  CAN FD Unpack/1 -> Data Type Conversion1/1
  CAN FD Unpack/2 -> Data Type Conversion2/1
  CAN FD Unpack/3 -> Data Type Conversion3/1
  CAN FD Unpack/4 -> Data Type Conversion4/1
  CAN FD Unpack/5 -> Data Type Conversion5/1
  CAN FD Unpack/6 -> Data Type Conversion6/1
  CAN FD Unpack/7 -> Data Type Conversion7/1
  Data Type Conversion1/1 -> Bus Creator/1  "IPM_ObjHeaderBlockCounter"
  Data Type Conversion2/1 -> Bus Creator/2  "IPM_ObjHeader_Checksum"
  Data Type Conversion3/1 -> Bus Creator/3  "IPM_ObjHeader_MsgCounter"
  Data Type Conversion4/1 -> Bus Creator/4  "IPM_Obj_TimeStampStatus"
  Data Type Conversion5/1 -> Bus Creator/5  "IPM_Obj_TimeStamp_Nsec"
  Data Type Conversion6/1 -> Bus Creator/6  "IPM_Obj_TimeStamp_sec"
  Data Type Conversion7/1 -> Bus Creator/7  "IPM_SensorState"
  Bus Creator/1 -> VR_ADCU_IPM_ObjHeader_0x630FromOutData/1  "VR_ADCU_IPM_ObjHeader_0x630FromOutData"
  VR_ADCU_IPM_ObjHeader_0x630FromInData/1 -> CAN FD Unpack/1  "VR_ADCU_IPM_ObjHeader_0x630FromInData"

== system ALL_JP360_DBW_V6_5_1103/MsgFromCAN/VR_ADCU_MsgFromCAN/VR_ADCU_IPM_Obj_01_0x650 ==
  VR_ADCU_IPM_Obj_01_0x650FromInData : Inport  OutDataTypeStr=Bus:CAN_FD_MESSAGE_BUS
  Bus Creator : BusCreator  Inputs=18  OutDataTypeStr=Bus:VR_ADCU_IPM_Obj_01_0x650  NonVirtualBus=on
  CAN FD Unpack : canfdmsglib/CAN FD Unpack  CANdbFile=HiFire_T360_P789_1R1V_Pri_Matrix_CAN_V2.3_20220810.dbc  MsgList=(none)  MsgName=IPM_Obj_01_0x650  ProtocolMode=CAN FD  MsgIDType=Standard (11-bit identifier)  MsgIdentifier=1616  MsgLength=32  SignalInfo={'IPM_ObjBlockCounter_01','13','11','BE','unsigned','Standard','0','1','0','0','2047';'IPM_ObjDistX_01','58','12','BE','unsigned','Standard','0','0.0625','0','0','254.9375';'IPM_ObjDistY_01','76','14','BE','unsigned','Standard','0','0.0078125','-64','-64','63.9922';'IPM_ObjID_01','16','8','BE','unsigned','Standard','0','1','0','0','255';'IPM_ObjRelAccelX_01','104','10','BE','unsigned','Standard','0','0.03125','-16','-16','15.9688';'IPM_ObjRelAccelY_01','126','10','BE','unsigned','Standard','0','0.03125','-16','-16','15.9688';'IPM_ObjRelVelX_01','95','13','BE','unsigned','Standard','0','0.03125','-128','-128','127.9688';'IPM_ObjRelVelY_01','98','13','BE','unsigned','Standard','0','0.03125','-128','-128','127.9688';'IPM_ObjType_01','54','4','BE','unsigned','Standard','0','1','0','0','15';'IPM_Obj_01_Checksum','248','16','BE','unsigned','Standard','0','1','0','0','65535';'IPM_Obj_01_MsgCounter','232','4','BE','unsigned','Standard','0','1','0','0','15';'IPM_Object_Age_01','37','11','BE','unsigned','Standard','0','1','0','0','2047';'IPM_Object_Existence_Probability_01','42','6','BE','unsigned','Standard','0','2','0','0','100';'IPM_Object_Heading_01','132','10','BE','unsigned','Standard','0','0.01','-3.14','-3.14','3.14';'IPM_Object_Height_01','167','9','BE','unsigned','Standard','0','0.01','0','0','5.11';'IPM_Object_Length_01','139','9','BE','unsigned','Standard','0','0.05','0','0','25.5';'IPM_Object_Motion_Status_01','161','3','BE','unsigned','Standard','0','1','0','0','7';'IPM_Object_Width_01','144','11','BE','unsigned','Standard','0','0.01','0','0','12'}  IDPort=off  TimestampPort=off  ErrorPort=off  RemotePort=off  LengthPort=off  StatusPort=off  BRSPort=off  ESIPort=off  DLCPort=off  ApplyMinMax=off
      settings: SourceProductBaseCode=ME,XP,VN  DataFormat=CANdb specified signals
  Data Type Conversion1 : DataTypeConversion  OutDataTypeStr=int16  SaturateOnIntegerOverflow=off  RndMeth=Floor
  Data Type Conversion10 : DataTypeConversion  OutDataTypeStr=uint16  SaturateOnIntegerOverflow=off  RndMeth=Floor
  Data Type Conversion{9,11,13,17} (4 alike) : DataTypeConversion  OutDataTypeStr=int8  SaturateOnIntegerOverflow=off  RndMeth=Floor
  Data Type Conversion12 : DataTypeConversion  OutDataTypeStr=int16  SaturateOnIntegerOverflow=off  RndMeth=Floor
  Data Type Conversion{2..3,5..8,14..16,18} (10 alike) : DataTypeConversion  OutDataTypeStr=single  SaturateOnIntegerOverflow=off  RndMeth=Floor
  Data Type Conversion4 : DataTypeConversion  OutDataTypeStr=uint8  SaturateOnIntegerOverflow=off  RndMeth=Floor
  VR_ADCU_IPM_Obj_01_0x650FromOutData : Outport  OutDataTypeStr=Bus:VR_ADCU_IPM_Obj_01_0x650
  wires:
  CAN FD Unpack/1 -> Data Type Conversion1/1
  CAN FD Unpack/2 -> Data Type Conversion2/1
  CAN FD Unpack/3 -> Data Type Conversion3/1
  CAN FD Unpack/4 -> Data Type Conversion4/1
  CAN FD Unpack/5 -> Data Type Conversion5/1
  CAN FD Unpack/6 -> Data Type Conversion6/1
  CAN FD Unpack/7 -> Data Type Conversion7/1
  CAN FD Unpack/8 -> Data Type Conversion8/1
  CAN FD Unpack/9 -> Data Type Conversion9/1
  CAN FD Unpack/10 -> Data Type Conversion10/1
  CAN FD Unpack/11 -> Data Type Conversion11/1
  CAN FD Unpack/12 -> Data Type Conversion12/1
  CAN FD Unpack/13 -> Data Type Conversion13/1
  CAN FD Unpack/14 -> Data Type Conversion14/1
  CAN FD Unpack/15 -> Data Type Conversion15/1
  CAN FD Unpack/16 -> Data Type Conversion16/1
  CAN FD Unpack/17 -> Data Type Conversion17/1
  CAN FD Unpack/18 -> Data Type Conversion18/1
  Data Type Conversion1/1 -> Bus Creator/1  "IPM_ObjBlockCounter_01"
  Data Type Conversion2/1 -> Bus Creator/2  "IPM_ObjDistX_01"
  Data Type Conversion3/1 -> Bus Creator/3  "IPM_ObjDistY_01"
  Data Type Conversion4/1 -> Bus Creator/4  "IPM_ObjID_01"
  Data Type Conversion5/1 -> Bus Creator/5  "IPM_ObjRelAccelX_01"
  Data Type Conversion6/1 -> Bus Creator/6  "IPM_ObjRelAccelY_01"
  Data Type Conversion7/1 -> Bus Creator/7  "IPM_ObjRelVelX_01"
  Data Type Conversion8/1 -> Bus Creator/8  "IPM_ObjRelVelY_01"
  Data Type Conversion9/1 -> Bus Creator/9  "IPM_ObjType_01"
  Data Type Conversion10/1 -> Bus Creator/10  "IPM_Obj_01_Checksum"
  Data Type Conversion11/1 -> Bus Creator/11  "IPM_Obj_01_MsgCounter"
  Data Type Conversion12/1 -> Bus Creator/12  "IPM_Object_Age_01"
  Data Type Conversion13/1 -> Bus Creator/13  "IPM_Object_Existence_Probability_01"
  Data Type Conversion14/1 -> Bus Creator/14  "IPM_Object_Heading_01"
  Data Type Conversion15/1 -> Bus Creator/15  "IPM_Object_Height_01"
  Data Type Conversion16/1 -> Bus Creator/16  "IPM_Object_Length_01"
  Data Type Conversion17/1 -> Bus Creator/17  "IPM_Object_Motion_Status_01"
  Data Type Conversion18/1 -> Bus Creator/18  "IPM_Object_Width_01"
  Bus Creator/1 -> VR_ADCU_IPM_Obj_01_0x650FromOutData/1  "VR_ADCU_IPM_Obj_01_0x650FromOutData"
  VR_ADCU_IPM_Obj_01_0x650FromInData/1 -> CAN FD Unpack/1  "VR_ADCU_IPM_Obj_01_0x650FromInData"

== system ALL_JP360_DBW_V6_5_1103/MsgFromCAN/VR_ADCU_MsgFromCAN/VR_ADCU_IPM_Obj_02_0x651 ==
  VR_ADCU_IPM_Obj_02_0x651FromInData : Inport  OutDataTypeStr=Bus:CAN_FD_MESSAGE_BUS
  Bus Creator : BusCreator  Inputs=18  OutDataTypeStr=Bus:VR_ADCU_IPM_Obj_02_0x651  NonVirtualBus=on
  CAN FD Unpack : canfdmsglib/CAN FD Unpack  CANdbFile=HiFire_T360_P789_1R1V_Pri_Matrix_CAN_V2.3_20220810.dbc  MsgList=(none)  MsgName=IPM_Obj_02_0x651  ProtocolMode=CAN FD  MsgIDType=Standard (11-bit identifier)  MsgIdentifier=1617  MsgLength=32  SignalInfo={'IPM_ObjBlockCounter_02','13','11','BE','unsigned','Standard','0','1','0','0','2047';'IPM_ObjDistX_02','58','12','BE','unsigned','Standard','0','0.0625','0','0','254.9375';'IPM_ObjDistY_02','76','14','BE','unsigned','Standard','0','0.0078125','-64','-64','63.9922';'IPM_ObjID_02','16','8','BE','unsigned','Standard','0','1','0','0','255';'IPM_ObjRelAccelX_02','104','10','BE','unsigned','Standard','0','0.03125','-16','-16','15.9688';'IPM_ObjRelAccelY_02','126','10','BE','unsigned','Standard','0','0.03125','-16','-16','15.9688';'IPM_ObjRelVelX_02','95','13','BE','unsigned','Standard','0','0.03125','-128','-128','127.9688';'IPM_ObjRelVelY_02','98','13','BE','unsigned','Standard','0','0.03125','-128','-128','127.9688';'IPM_ObjType_02','54','4','BE','unsigned','Standard','0','1','0','0','15';'IPM_Obj_02_Checksum','248','16','BE','unsigned','Standard','0','1','0','0','65535';'IPM_Obj_02_MsgCounter','232','4','BE','unsigned','Standard','0','1','0','0','15';'IPM_Object_Age_02','37','11','BE','unsigned','Standard','0','1','0','0','2047';'IPM_Object_Existence_Probability_02','42','6','BE','unsigned','Standard','0','2','0','0','100';'IPM_Object_Heading_02','132','10','BE','unsigned','Standard','0','0.01','-3.14','-3.14','3.14';'IPM_Object_Height_02','167','9','BE','unsigned','Standard','0','0.01','0','0','5.11';'IPM_Object_Length_02','139','9','BE','unsigned','Standard','0','0.05','0','0','25.5';'IPM_Object_Motion_Status_02','161','3','BE','unsigned','Standard','0','1','0','0','7';'IPM_Object_Width_02','144','11','BE','unsigned','Standard','0','0.01','0','0','12'}  IDPort=off  TimestampPort=off  ErrorPort=off  RemotePort=off  LengthPort=off  StatusPort=off  BRSPort=off  ESIPort=off  DLCPort=off  ApplyMinMax=off
      settings: SourceProductBaseCode=ME,XP,VN  DataFormat=CANdb specified signals
  Data Type Conversion1 : DataTypeConversion  OutDataTypeStr=int16  SaturateOnIntegerOverflow=off  RndMeth=Floor
  Data Type Conversion10 : DataTypeConversion  OutDataTypeStr=uint16  SaturateOnIntegerOverflow=off  RndMeth=Floor
  Data Type Conversion{9,11,13,17} (4 alike) : DataTypeConversion  OutDataTypeStr=int8  SaturateOnIntegerOverflow=off  RndMeth=Floor
  Data Type Conversion12 : DataTypeConversion  OutDataTypeStr=int16  SaturateOnIntegerOverflow=off  RndMeth=Floor
  Data Type Conversion{2..3,5..8,14..16,18} (10 alike) : DataTypeConversion  OutDataTypeStr=single  SaturateOnIntegerOverflow=off  RndMeth=Floor
  Data Type Conversion4 : DataTypeConversion  OutDataTypeStr=uint8  SaturateOnIntegerOverflow=off  RndMeth=Floor
  VR_ADCU_IPM_Obj_02_0x651FromOutData : Outport  OutDataTypeStr=Bus:VR_ADCU_IPM_Obj_02_0x651
  wires:
  CAN FD Unpack/1 -> Data Type Conversion1/1
  CAN FD Unpack/2 -> Data Type Conversion2/1
  CAN FD Unpack/3 -> Data Type Conversion3/1
  CAN FD Unpack/4 -> Data Type Conversion4/1
  CAN FD Unpack/5 -> Data Type Conversion5/1
  CAN FD Unpack/6 -> Data Type Conversion6/1
  CAN FD Unpack/7 -> Data Type Conversion7/1
  CAN FD Unpack/8 -> Data Type Conversion8/1
  CAN FD Unpack/9 -> Data Type Conversion9/1
  CAN FD Unpack/10 -> Data Type Conversion10/1
  CAN FD Unpack/11 -> Data Type Conversion11/1
  CAN FD Unpack/12 -> Data Type Conversion12/1
  CAN FD Unpack/13 -> Data Type Conversion13/1
  CAN FD Unpack/14 -> Data Type Conversion14/1
  CAN FD Unpack/15 -> Data Type Conversion15/1
  CAN FD Unpack/16 -> Data Type Conversion16/1
  CAN FD Unpack/17 -> Data Type Conversion17/1
  CAN FD Unpack/18 -> Data Type Conversion18/1
  Data Type Conversion1/1 -> Bus Creator/1  "IPM_ObjBlockCounter_02"
  Data Type Conversion2/1 -> Bus Creator/2  "IPM_ObjDistX_02"
  Data Type Conversion3/1 -> Bus Creator/3  "IPM_ObjDistY_02"
  Data Type Conversion4/1 -> Bus Creator/4  "IPM_ObjID_02"
  Data Type Conversion5/1 -> Bus Creator/5  "IPM_ObjRelAccelX_02"
  Data Type Conversion6/1 -> Bus Creator/6  "IPM_ObjRelAccelY_02"
  Data Type Conversion7/1 -> Bus Creator/7  "IPM_ObjRelVelX_02"
  Data Type Conversion8/1 -> Bus Creator/8  "IPM_ObjRelVelY_02"
  Data Type Conversion9/1 -> Bus Creator/9  "IPM_ObjType_02"
  Data Type Conversion10/1 -> Bus Creator/10  "IPM_Obj_02_Checksum"
  Data Type Conversion11/1 -> Bus Creator/11  "IPM_Obj_02_MsgCounter"
  Data Type Conversion12/1 -> Bus Creator/12  "IPM_Object_Age_02"
  Data Type Conversion13/1 -> Bus Creator/13  "IPM_Object_Existence_Probability_02"
  Data Type Conversion14/1 -> Bus Creator/14  "IPM_Object_Heading_02"
  Data Type Conversion15/1 -> Bus Creator/15  "IPM_Object_Height_02"
  Data Type Conversion16/1 -> Bus Creator/16  "IPM_Object_Length_02"
  Data Type Conversion17/1 -> Bus Creator/17  "IPM_Object_Motion_Status_02"
  Data Type Conversion18/1 -> Bus Creator/18  "IPM_Object_Width_02"
  Bus Creator/1 -> VR_ADCU_IPM_Obj_02_0x651FromOutData/1  "VR_ADCU_IPM_Obj_02_0x651FromOutData"
  VR_ADCU_IPM_Obj_02_0x651FromInData/1 -> CAN FD Unpack/1  "VR_ADCU_IPM_Obj_02_0x651FromInData"

== system ALL_JP360_DBW_V6_5_1103/MsgFromCAN/VR_ADCU_MsgFromCAN/VR_ADCU_IPM_Obj_03_0x652 ==
  VR_ADCU_IPM_Obj_03_0x652FromInData : Inport  OutDataTypeStr=Bus:CAN_FD_MESSAGE_BUS
  Bus Creator : BusCreator  Inputs=18  OutDataTypeStr=Bus:VR_ADCU_IPM_Obj_03_0x652  NonVirtualBus=on
  CAN FD Unpack : canfdmsglib/CAN FD Unpack  CANdbFile=HiFire_T360_P789_1R1V_Pri_Matrix_CAN_V2.3_20220810.dbc  MsgList=(none)  MsgName=IPM_Obj_03_0x652  ProtocolMode=CAN FD  MsgIDType=Standard (11-bit identifier)  MsgIdentifier=1618  MsgLength=32  SignalInfo={'IPM_ObjBlockCounter_03','13','11','BE','unsigned','Standard','0','1','0','0','2047';'IPM_ObjDistX_03','58','12','BE','unsigned','Standard','0','0.0625','0','0','254.9375';'IPM_ObjDistY_03','76','14','BE','unsigned','Standard','0','0.0078125','-64','-64','63.9922';'IPM_ObjID_03','16','8','BE','unsigned','Standard','0','1','0','0','255';'IPM_ObjRelAccelX_03','104','10','BE','unsigned','Standard','0','0.03125','-16','-16','15.9688';'IPM_ObjRelAccelY_03','126','10','BE','unsigned','Standard','0','0.03125','-16','-16','15.9688';'IPM_ObjRelVelX_03','95','13','BE','unsigned','Standard','0','0.03125','-128','-128','127.9688';'IPM_ObjRelVelY_03','98','13','BE','unsigned','Standard','0','0.03125','-128','-128','127.9688';'IPM_ObjType_03','54','4','BE','unsigned','Standard','0','1','0','0','15';'IPM_Obj_03_Checksum','248','16','BE','unsigned','Standard','0','1','0','0','65535';'IPM_Obj_03_MsgCounter','232','4','BE','unsigned','Standard','0','1','0','0','15';'IPM_Object_Age_03','37','11','BE','unsigned','Standard','0','1','0','0','2047';'IPM_Object_Existence_Probability_03','42','6','BE','unsigned','Standard','0','2','0','0','100';'IPM_Object_Heading_03','132','10','BE','unsigned','Standard','0','0.01','-3.14','-3.14','3.14';'IPM_Object_Height_03','167','9','BE','unsigned','Standard','0','0.01','0','0','5.11';'IPM_Object_Length_03','139','9','BE','unsigned','Standard','0','0.05','0','0','25.5';'IPM_Object_Motion_Status_03','161','3','BE','unsigned','Standard','0','1','0','0','7';'IPM_Object_Width_03','144','11','BE','unsigned','Standard','0','0.01','0','0','12'}  IDPort=off  TimestampPort=off  ErrorPort=off  RemotePort=off  LengthPort=off  StatusPort=off  BRSPort=off  ESIPort=off  DLCPort=off  ApplyMinMax=off
      settings: SourceProductBaseCode=ME,XP,VN  DataFormat=CANdb specified signals
  Data Type Conversion1 : DataTypeConversion  OutDataTypeStr=int16  SaturateOnIntegerOverflow=off  RndMeth=Floor
  Data Type Conversion10 : DataTypeConversion  OutDataTypeStr=uint16  SaturateOnIntegerOverflow=off  RndMeth=Floor
  Data Type Conversion{9,11,13,17} (4 alike) : DataTypeConversion  OutDataTypeStr=int8  SaturateOnIntegerOverflow=off  RndMeth=Floor
  Data Type Conversion12 : DataTypeConversion  OutDataTypeStr=int16  SaturateOnIntegerOverflow=off  RndMeth=Floor
  Data Type Conversion{2..3,5..8,14..16,18} (10 alike) : DataTypeConversion  OutDataTypeStr=single  SaturateOnIntegerOverflow=off  RndMeth=Floor
  Data Type Conversion4 : DataTypeConversion  OutDataTypeStr=uint8  SaturateOnIntegerOverflow=off  RndMeth=Floor
  VR_ADCU_IPM_Obj_03_0x652FromOutData : Outport  OutDataTypeStr=Bus:VR_ADCU_IPM_Obj_03_0x652
  wires:
  CAN FD Unpack/1 -> Data Type Conversion1/1
  CAN FD Unpack/2 -> Data Type Conversion2/1
  CAN FD Unpack/3 -> Data Type Conversion3/1
  CAN FD Unpack/4 -> Data Type Conversion4/1
  CAN FD Unpack/5 -> Data Type Conversion5/1
  CAN FD Unpack/6 -> Data Type Conversion6/1
  CAN FD Unpack/7 -> Data Type Conversion7/1
  CAN FD Unpack/8 -> Data Type Conversion8/1
  CAN FD Unpack/9 -> Data Type Conversion9/1
  CAN FD Unpack/10 -> Data Type Conversion10/1
  CAN FD Unpack/11 -> Data Type Conversion11/1
  CAN FD Unpack/12 -> Data Type Conversion12/1
  CAN FD Unpack/13 -> Data Type Conversion13/1
  CAN FD Unpack/14 -> Data Type Conversion14/1
  CAN FD Unpack/15 -> Data Type Conversion15/1
  CAN FD Unpack/16 -> Data Type Conversion16/1
  CAN FD Unpack/17 -> Data Type Conversion17/1
  CAN FD Unpack/18 -> Data Type Conversion18/1
  Data Type Conversion1/1 -> Bus Creator/1  "IPM_ObjBlockCounter_03"
  Data Type Conversion2/1 -> Bus Creator/2  "IPM_ObjDistX_03"
  Data Type Conversion3/1 -> Bus Creator/3  "IPM_ObjDistY_03"
  Data Type Conversion4/1 -> Bus Creator/4  "IPM_ObjID_03"
  Data Type Conversion5/1 -> Bus Creator/5  "IPM_ObjRelAccelX_03"
  Data Type Conversion6/1 -> Bus Creator/6  "IPM_ObjRelAccelY_03"
  Data Type Conversion7/1 -> Bus Creator/7  "IPM_ObjRelVelX_03"
  Data Type Conversion8/1 -> Bus Creator/8  "IPM_ObjRelVelY_03"
  Data Type Conversion9/1 -> Bus Creator/9  "IPM_ObjType_03"
  Data Type Conversion10/1 -> Bus Creator/10  "IPM_Obj_03_Checksum"
  Data Type Conversion11/1 -> Bus Creator/11  "IPM_Obj_03_MsgCounter"
  Data Type Conversion12/1 -> Bus Creator/12  "IPM_Object_Age_03"
  Data Type Conversion13/1 -> Bus Creator/13  "IPM_Object_Existence_Probability_03"
  Data Type Conversion14/1 -> Bus Creator/14  "IPM_Object_Heading_03"
  Data Type Conversion15/1 -> Bus Creator/15  "IPM_Object_Height_03"
  Data Type Conversion16/1 -> Bus Creator/16  "IPM_Object_Length_03"
  Data Type Conversion17/1 -> Bus Creator/17  "IPM_Object_Motion_Status_03"
  Data Type Conversion18/1 -> Bus Creator/18  "IPM_Object_Width_03"
  Bus Creator/1 -> VR_ADCU_IPM_Obj_03_0x652FromOutData/1  "VR_ADCU_IPM_Obj_03_0x652FromOutData"
  VR_ADCU_IPM_Obj_03_0x652FromInData/1 -> CAN FD Unpack/1  "VR_ADCU_IPM_Obj_03_0x652FromInData"
